simulink subsystem "ZOH_Regulator"  (R2023a)
settings: Solver=VariableStepAuto  StartTime=0.0  StopTime=10.0  RelTol=1e-3
settings Model: Creator=user  LastModifiedBy=user

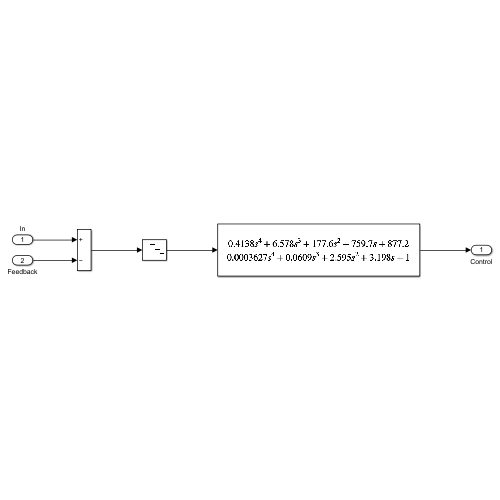
[thumbnail: Simulink's stored preview of the top-level diagram]
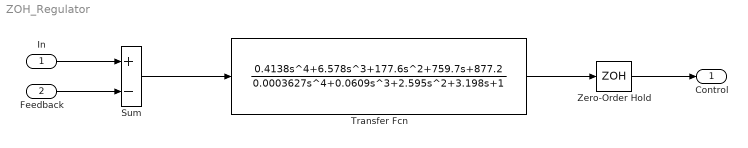
== system ZOH_Regulator ==
  In : Inport
  Feedback : Inport  Port=2
  Sum : Sum  Inputs=+-
  Transfer Fcn : TransferFcn  Numerator=[0.4138, 6.578, 177.6, 759.7, 877.2]  Denominator=[0.0003627, 0.0609, 2.595, 3.198 1]
  Zero-Order Hold : ZeroOrderHold  SampleTime=0.005
  Control : Outport
  wires:
  Sum/1 -> Transfer Fcn/1
  In/1 -> Sum/1
  Feedback/1 -> Sum/2
  Transfer Fcn/1 -> Zero-Order Hold/1
  Zero-Order Hold/1 -> Control/1
